simulink model "control_PID"  (R2018a)
settings: Solver=VariableStepAuto  StartTime=0.0  StopTime=300  MaxStep=0.05  RelTol=1e-3
values from neighbouring files (symbols this model uses):
  ro = 0.0683    [LaplaceAzeta.m]    (also in discretizacion.m = 0.0683238685925)
  so = 0.3356    [LaplaceAzeta.m]    (also in discretizacion.m = 0.335599308431)
  uo = 0.12    [LaplaceAzeta.m]    (also in discretizacion.m)
undefined symbols (not defined in the file or in its folder): kp, td, ti
libraries: simulink x6
settings Model: Creator=posoriol1  LastModifiedBy=posoriol1
settings CodeAppCC: StateflowObjectComments=on

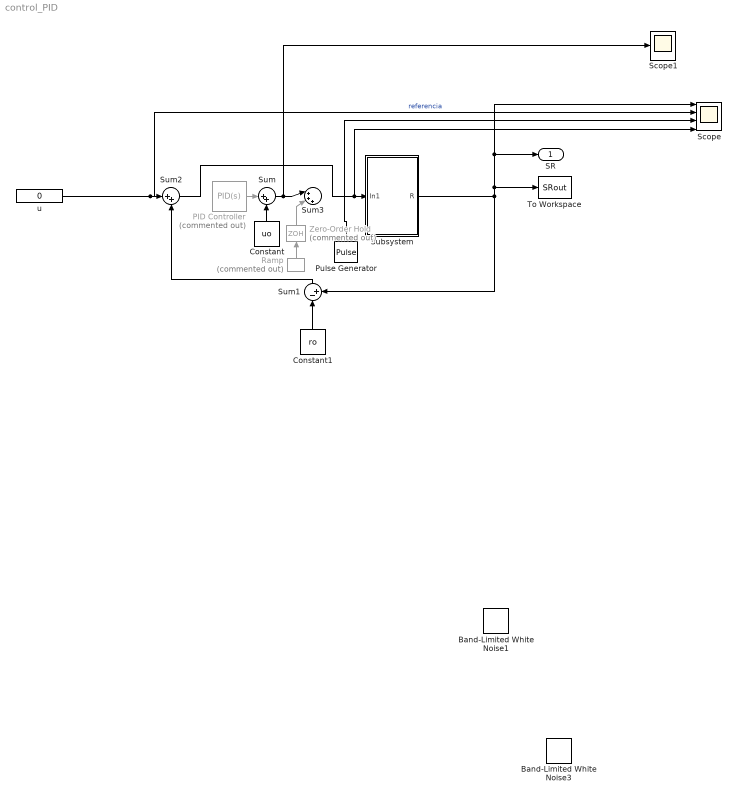
== system control_PID ==
  Band-Limited White Noise1 : simulink/Sources/Band-Limited White Noise  Cov=[0.0000005]  Ts=0.3  seed=[11558]
  Band-Limited White Noise3 : simulink/Sources/Band-Limited White Noise  Cov=[0.0000005]  Ts=0.3  seed=[11558]
  Constant : Constant  Value=uo
  Constant1 : Constant  Value=ro
  PID Controller : simulink/Continuous/PID Controller  Commented=on  Controller=PID  TimeDomain=Continuous-time  SampleTime=-1  IntegratorMethod=Forward Euler  FilterMethod=Forward Euler  Form=Parallel  UseFilter=on  ControllerParametersSource=internal  P=kp  I=kp/ti  D=kp*td  N=100  InitialConditionSource=internal  InitialConditionForIntegrator=0  InitialConditionForFilter=0  ExternalReset=none  LimitOutput=off  UpperSaturationLimit=inf  LowerSaturationLimit=-inf  LinearizeAsGain=on  AntiWindupMode=none  Kb=1  TrackingMode=off  Kt=1  PParamMin=[]  PParamMax=[]  IParamMin=[]  IParamMax=[]  DParamMin=[]  DParamMax=[]  NParamMin=[]  NParamMax=[]  KbParamMin=[]  KbParamMax=[]  KtParamMin=[]  KtParamMax=[]  POutMin=[]  POutMax=[]  IOutMin=[]  IOutMax=[]  DOutMin=[]  DOutMax=[]  NOutMin=[]  NOutMax=[]  KbOutMin=[]  KbOutMax=[]  KtOutMin=[]  KtOutMax=[]  IntegratorOutMin=[]  IntegratorOutMax=[]  FilterOutMin=[]  FilterOutMax=[]  SumOutMin=[]  SumOutMax=[]  SumI1OutMin=[]  SumI1OutMax=[]  SumI2OutMin=[]  SumI2OutMax=[]  SumI3OutMin=[]  SumI3OutMax=[]  SumDOutMin=[]  SumDOutMax=[]  SaturationOutMin=[]  SaturationOutMax=[]  IntegratorContinuousStateAttributes=''  IntegratorStateMustResolveToSignalObject=off  IntegratorRTWStateStorageClass=Auto  FilterContinuousStateAttributes=''  FilterStateMustResolveToSignalObject=off  FilterRTWStateStorageClass=Auto  DifferentiatorICPrevScaledInput=0  DifferentiatorOutMin=[]  DifferentiatorOutMax=[]  FilterDiffOutCoefMin=[]  FilterDiffOutCoefMax=[]  SumDenOutMin=[]  SumDenOutMax=[]  SumNumOutMin=[]  SumNumOutMax=[]  ReciprocalOutMin=[]  ReciprocalOutMax=[]  DivideOutMin=[]  DivideOutMax=[]  TunerSelectOption=Transfer Function Based (PID Tuner App)
  Pulse Generator : DiscretePulseGenerator  PulseType=Time based  Period=10  PulseWidth=5
  Ramp : simulink/Sources/Ramp  Commented=on  slope=0.4/300  start=0  InitialOutput=0
  Scope : Scope  NumInputPorts=4
  Scope1 : Scope
  Subsystem : Subsystem  mask{par=[0.14 0.1 0.3960 4^(-3) 0.2 0.09 0.0083], x0=[so, ro]}
      mask prompts: par "[bs br alphas q ms mr mc]"; x0 "Cond iniciales (s0,r0)"
      mask init:
      | bs=par(1);br=par(2);alphas=par(3);q=par(4);ms=par(5);mr=par(6);mc=par(7);
  Sum : Sum  Inputs=|++
  Sum1 : Sum  Inputs=|-+
  Sum2 : Sum  Inputs=|++
  Sum3 : Sum  Inputs=|+++
  To Workspace : ToWorkspace  VariableName=SRout  SampleTime=-1
  Zero-Order Hold : ZeroOrderHold  Commented=on  SampleTime=40
  u : Constant  Value=0
  SR : Outport
  wires:
  PID Controller/1 -> Sum/1
  Constant/1 -> Sum/2
  Sum/1 -> Scope1/1, Sum3/1
  u/1 -> Sum2/1, Scope/2  "referencia"
  Subsystem/1(R) -> SR/1, Scope/1, To Workspace/1, Sum1/2
  Constant1/1 -> Sum1/1
  Sum1/1 -> Sum2/2
  Sum2/1 -> Scope/4, Subsystem/1(In1)
  Pulse Generator/1 -> Scope/3
  Ramp/1 -> Zero-Order Hold/1
  Zero-Order Hold/1 -> Sum3/2

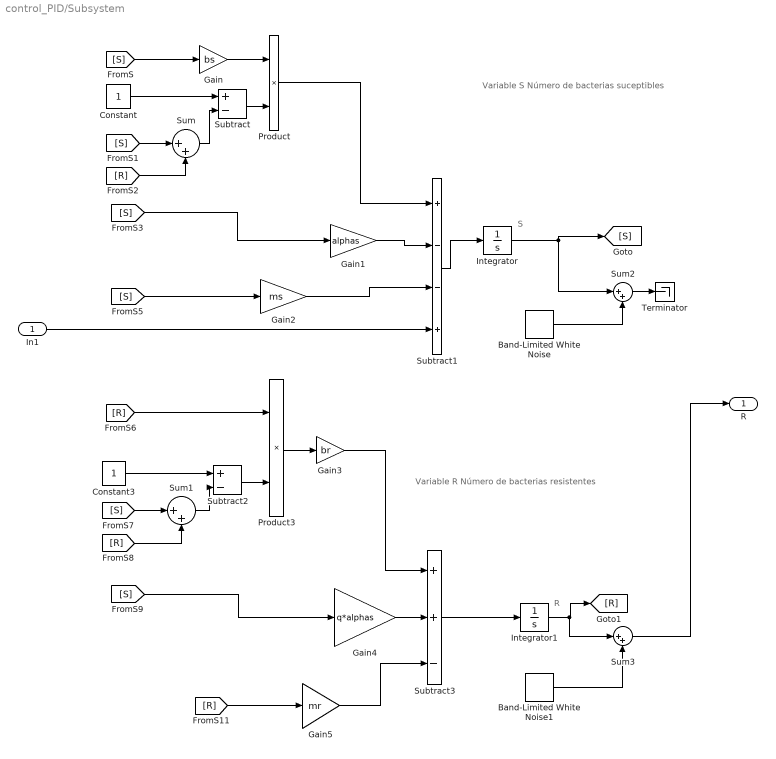
== system control_PID/Subsystem ==
  note: R
  note: S
  note: Variable S
      | Número de bacterias suceptibles
  note: Variable R
      | Número de bacterias resistentes
  In1 : Inport
  Band-Limited White Noise : simulink/Sources/Band-Limited White Noise  Cov=[0.000001/100]  Ts=0.3  seed=[23341]
  Band-Limited White Noise1 : simulink/Sources/Band-Limited White Noise  Cov=[0.0000005/100]  Ts=0.3  seed=[11558]
  Constant : Constant
  Constant3 : Constant
  Gain : Gain  Gain=bs
  Gain1 : Gain  Gain=alphas
  Gain2 : Gain  Gain=ms
  Gain3 : Gain  Gain=br
  Gain4 : Gain  Gain=q*alphas
  Gain5 : Gain  Gain=mr
  Integrator : Integrator  InitialCondition=x0(1)
  Integrator1 : Integrator  InitialCondition=x0(2)
  Product : Product
  Product3 : Product
  Subtract : Sum  Inputs=+-
  Subtract1 : Sum  Inputs=+--+
  Subtract2 : Sum  Inputs=+-
  Subtract3 : Sum  Inputs=++-
  Sum{,1..3} (4 alike) : Sum  Inputs=|++
  Terminator : Terminator
  R : Outport
  wires:
  [S] -> Sum/1
  [R] -> Sum/2
  Constant/1 -> Subtract/1
  [S] -> Sum1/1
  Sum1/1 -> Subtract2/2
  Subtract1/1 -> Integrator/1
  Integrator/1 -> [S], Sum2/1
  [R] -> Sum1/2
  Constant3/1 -> Subtract2/1
  Product3/1 -> Gain3/1
  Product/1 -> Subtract1/1
  Integrator1/1 -> Sum3/1, [R]
  Subtract3/1 -> Integrator1/1
  Sum/1 -> Subtract/2
  [S] -> Gain/1
  Gain/1 -> Product/1
  Subtract/1 -> Product/2
  [S] -> Gain1/1
  Gain1/1 -> Subtract1/2
  [S] -> Gain2/1
  Gain2/1 -> Subtract1/3
  Gain3/1 -> Subtract3/1
  [R] -> Product3/1
  Subtract2/1 -> Product3/2
  Gain4/1 -> Subtract3/2
  [S] -> Gain4/1
  Gain5/1 -> Subtract3/3
  [R] -> Gain5/1
  In1/1 -> Subtract1/4
  Band-Limited White Noise/1 -> Sum2/2
  Band-Limited White Noise1/1 -> Sum3/2
  Sum3/1 -> R/1
  Sum2/1 -> Terminator/1
